simulink model "BaB_RL_V8"  (R2021a)
settings: Solver=VariableStepAuto  StartTime=0.0  StopTime=10  RelTol=1e-3
undefined symbols (not defined in the file or in its folder): sensor, theory
libraries: simulink x2, rllib x1
settings Model: Creator=austinberg  LastModifiedBy=austinberg
settings SolverCC: ZeroCrossAlgorithm=Adaptive
settings DebuggingCC: MaskedZcDiagnostic=none  IgnoredZcDiagnostic=none

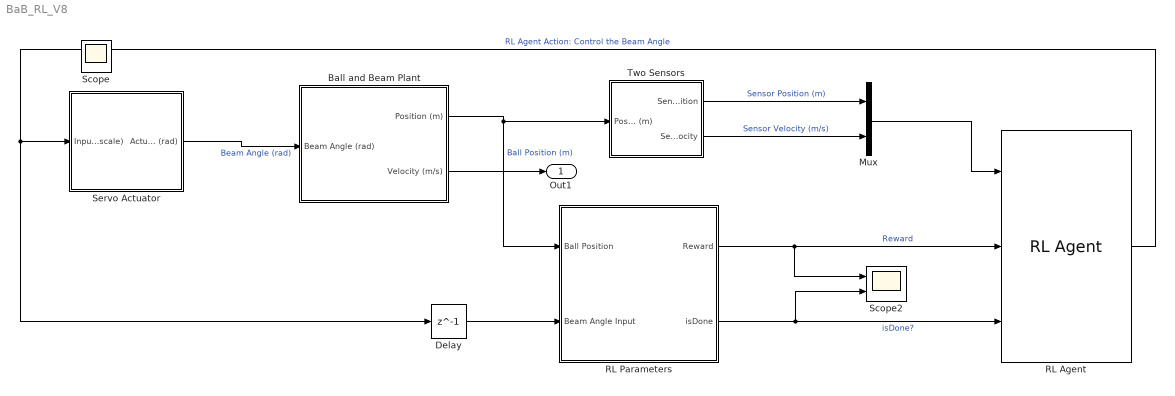
== system BaB_RL_V8 ==
  Ball and Beam Plant : Subsystem
      mask Display: image('PlantImage.png'); % Use "Edit Image" on toolstrip to change.
  Delay : Delay  DelayLength=1
  Mux : Mux  Inputs=2
  RL Agent : rllib/RL Agent  Agent=agent  ExternalActionAsInput=off  ProvideCumRwd=off  TreatAsDirectFeedthrough=on
  RL Parameters : Subsystem
  Scope2 : Scope  NumInputPorts=2
  Servo Actuator : Subsystem
      mask Display: image('servo.png'); % Use "Edit Image" on toolstrip to change.
  Two Sensors : Subsystem
      mask Display: image('Sensor.jpeg'); % Use "Edit Image" on toolstrip to change.
  Out1 : Outport
  Scope : Scope
  wires:
  Servo Actuator/1(Actual Beam Angle (rad)) -> Ball and Beam Plant/1(Beam Angle (rad))  "Beam Angle (rad)"
  Ball and Beam Plant/1(Position (m)) -> RL Parameters/1(Ball Position), Two Sensors/1(Position (m))  "Ball Position (m)"
  RL Parameters/1(Reward) -> RL Agent/2, Scope2/1  "Reward"
  Mux/1 -> RL Agent/1
  RL Parameters/2(isDone) -> RL Agent/3, Scope2/2  "isDone?"
  Two Sensors/1(Sensor Position) -> Mux/1  "Sensor Position (m)"
  Two Sensors/2(Sensor Velocity) -> Mux/2  "Sensor Velocity (m/s)"
  RL Agent/1 -> Delay/1, Servo Actuator/1(Input Angle (0-1 scale))  "RL Agent Action: Control the Beam Angle"
  Delay/1 -> RL Parameters/2(Beam Angle Input)
  Ball and Beam Plant/2(Velocity (m/s)) -> Out1/1

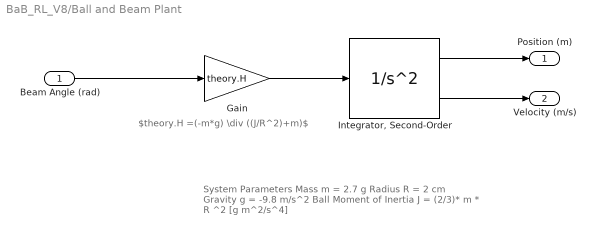
== system BaB_RL_V8/Ball and Beam Plant ==
  note: $theory.H =(-m*g) \div ((J/R^2)+m)$
  note: System Parameters
      |
      | Mass m = 2.7 g
      | Radius R = 2 cm
      | Gravity g = -9.8 m/s^2
      | Ball Moment of Inertia J = (2/3)* m * R ^2 [g m^2/s^4]
  Beam Angle (rad) : Inport
  Gain : Gain  Gain=theory.H
  "Integrator, Second-Order " : SecondOrderIntegrator  ICX=IC  LimitX=on  UpperLimitX=0.28  LowerLimitX=-0.28
  Position (m) : Outport
  Velocity (m/s) : Outport  Port=2
  wires:
  Beam Angle (rad)/1 -> Gain/1
  "Integrator, Second-Order "/1 -> Position (m)/1
  Gain/1 -> "Integrator, Second-Order "/1
  "Integrator, Second-Order "/2 -> Velocity (m/s)/1

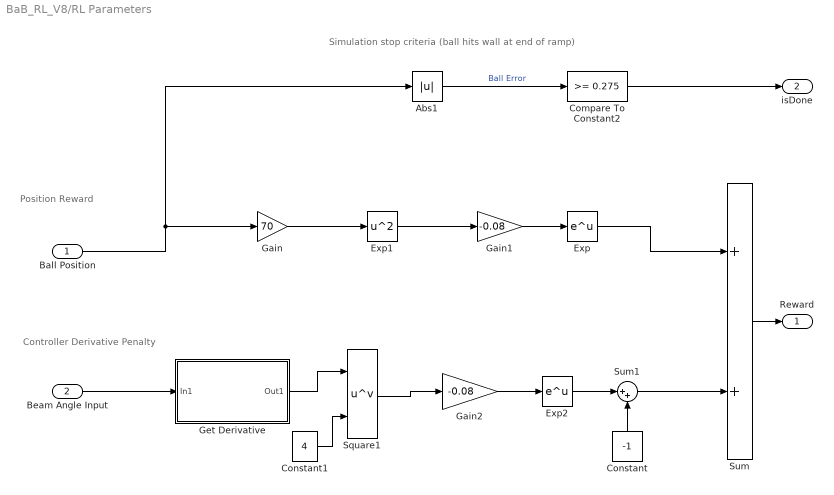
== system BaB_RL_V8/RL Parameters ==
  note: Controller Derivative Penalty
  note: Position Reward
  note: Simulation stop criteria (ball hits wall at end of ramp)
  Ball Position : Inport
  Beam Angle Input : Inport  Port=2
  Abs1 : Abs
  Compare To Constant2 : simulink/Logic and Bit Operations/Compare To Constant  relop=>=  const=0.275  OutDataTypeStr=boolean
  Constant : Constant  Value=-1
  Constant1 : Constant  Value=4
  Exp : Math  SaturateOnIntegerOverflow=on
  Exp1 : Math  Operator=square  SaturateOnIntegerOverflow=on
  Exp2 : Math  SaturateOnIntegerOverflow=on
  Gain : Gain  Gain=70
  Gain1 : Gain  Gain=-0.08
  Gain2 : Gain  Gain=-0.08
  Get Derivative : Subsystem
  Square1 : Math  Operator=pow  SaturateOnIntegerOverflow=on
  Sum : Sum
  Sum1 : Sum  Inputs=|++
  Reward : Outport
  isDone : Outport  Port=2
  wires:
  Abs1/1 -> Compare To Constant2/1  "Ball Error"
  Ball Position/1 -> Gain/1, Abs1/1
  Compare To Constant2/1 -> isDone/1
  Gain/1 -> Exp1/1
  Sum/1 -> Reward/1
  Exp1/1 -> Gain1/1
  Gain2/1 -> Exp2/1
  Get Derivative/1(Out1) -> Square1/1
  Square1/1 -> Gain2/1
  Exp2/1 -> Sum1/1
  Constant/1 -> Sum1/2
  Sum1/1 -> Sum/2
  Beam Angle Input/1 -> Get Derivative/1(In1)
  Gain1/1 -> Exp/1
  Exp/1 -> Sum/1
  Constant1/1 -> Square1/2

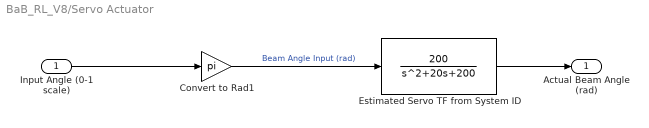
== system BaB_RL_V8/Servo Actuator ==
  Input Angle (0-1 scale) : Inport
  Convert to Rad1 : Gain  Gain=pi
  Estimated Servo TF from System ID : TransferFcn  Numerator=[0 0 200]  Denominator=[1 20 200]
  Actual Beam Angle (rad) : Outport
  wires:
  Convert to Rad1/1 -> Estimated Servo TF from System ID/1  "Beam Angle Input (rad)"
  Input Angle (0-1 scale)/1 -> Convert to Rad1/1
  Estimated Servo TF from System ID/1 -> Actual Beam Angle (rad)/1

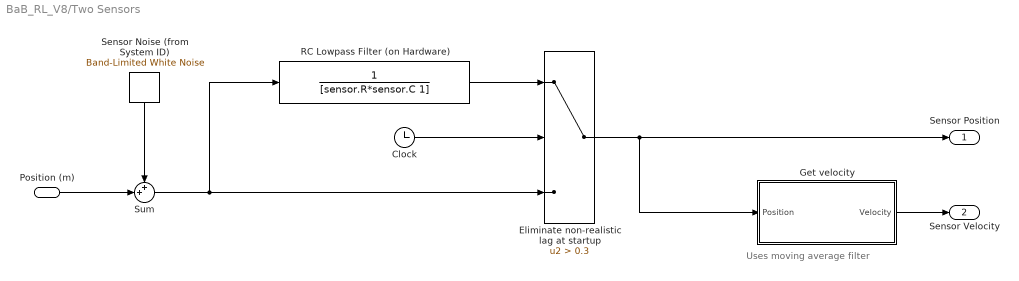
== system BaB_RL_V8/Two Sensors ==
  note: Uses moving average filter
  Position (m) : Inport
  Clock : Clock
  Eliminate non-realistic lag at startup : Switch  Criteria=u2 > Threshold  Threshold=0.3
  Get velocity : Subsystem
  RC Lowpass Filter (on Hardware) : TransferFcn  Denominator=[sensor.R*sensor.C 1]
  Sensor Noise (from System ID) : simulink/Sources/Band-Limited White Noise  Cov=sensor.NoisePower  Ts=sensor.SampleTime  seed=[23354]
  Sum : Sum  Inputs=++|
  Sensor Position : Outport
  Sensor Velocity : Outport  Port=2
  wires:
  Position (m)/1 -> Sum/2
  Sensor Noise (from System ID)/1 -> Sum/1
  Sum/1 -> RC Lowpass Filter (on Hardware)/1, Eliminate non-realistic lag at startup/3
  Clock/1 -> Eliminate non-realistic lag at startup/2
  RC Lowpass Filter (on Hardware)/1 -> Eliminate non-realistic lag at startup/1
  Eliminate non-realistic lag at startup/1 -> Sensor Position/1, Get velocity/1(Position)
  Get velocity/1(Velocity) -> Sensor Velocity/1

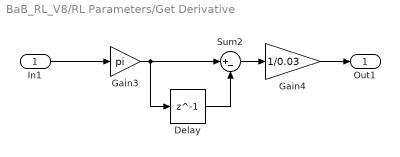
== system BaB_RL_V8/RL Parameters/Get Derivative ==
  In1 : Inport
  Delay : Delay  DelayLength=1
  Gain3 : Gain  Gain=pi
  Gain4 : Gain  Gain=1/0.03
  Sum2 : Sum  Inputs=|+-
  Out1 : Outport
  wires:
  In1/1 -> Gain3/1
  Gain4/1 -> Out1/1
  Delay/1 -> Sum2/2
  Sum2/1 -> Gain4/1
  Gain3/1 -> Delay/1, Sum2/1

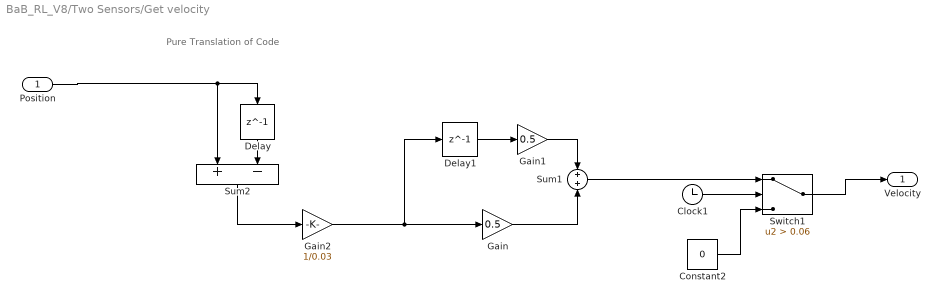
== system BaB_RL_V8/Two Sensors/Get velocity ==
  note: Pure Translation of Code
  Position : Inport
  Clock1 : Clock
  Constant2 : Constant  Value=0
  Delay : Delay  DelayLength=1
  Delay1 : Delay  DelayLength=1  SampleTime=0.03
  Gain : Gain  Gain=0.5
  Gain1 : Gain  Gain=0.5
  Gain2 : Gain  Gain=1/0.03
  Sum1 : Sum  Inputs=+|+
  Sum2 : Sum  Inputs=+-
  Switch1 : Switch  Criteria=u2 > Threshold  Threshold=0.06
  Velocity : Outport
  wires:
  Gain/1 -> Sum1/2
  Sum2/1 -> Gain2/1
  Switch1/1 -> Velocity/1
  Constant2/1 -> Switch1/3
  Position/1 -> Delay/1, Sum2/1
  Delay1/1 -> Gain1/1
  Clock1/1 -> Switch1/2
  Gain1/1 -> Sum1/1
  Delay/1 -> Sum2/2
  Gain2/1 -> Delay1/1, Gain/1
  Sum1/1 -> Switch1/1
